simulink model "sistema_nastro_trasportatore"  (R2017a)
settings: Solver=VariableStepAuto  StartTime=0.0  StopTime=10.0  RelTol=1e-3
values from neighbouring files (symbols this model uses):
  A = ro*area    (= 1500)    [params.m]
  B = Ks/A    (= 0.5)    [params.m]
  C = 1    [params.m]
  Km = 1/Y_MAX    (= 0.1)    [params.m]
  r = 0.5    [params.m]
  T = 0.1    [params.m]
  tau = 0.6    [params.m]
libraries: simulink x3
settings Model: Creator=Lucario95  LastModifiedBy=Lucario95

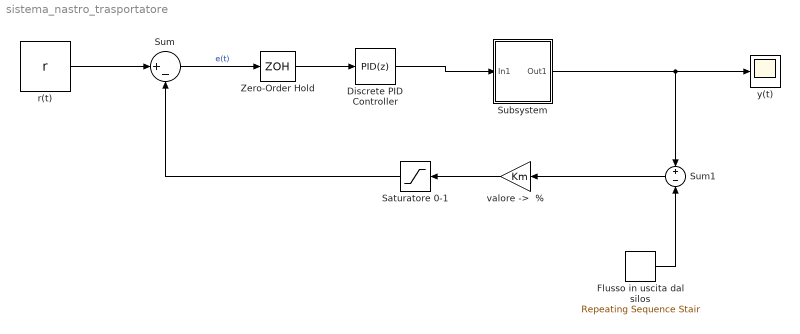
== system sistema_nastro_trasportatore ==
  Discrete PID Controller : simulink/Continuous/PID Controller  Controller=PID  TimeDomain=Discrete-time  SampleTime=-1  IntegratorMethod=Forward Euler  FilterMethod=Forward Euler  Form=Parallel  UseFilter=on  ControllerParametersSource=internal  P=1  I=1  D=0  N=100  InitialConditionSource=internal  InitialConditionForIntegrator=0  InitialConditionForFilter=0  ExternalReset=none  LimitOutput=off  UpperSaturationLimit=inf  LowerSaturationLimit=-inf  LinearizeAsGain=off  AntiWindupMode=none  Kb=1  TrackingMode=off  Kt=1  PParamMin=[]  PParamMax=[]  IParamMin=[]  IParamMax=[]  DParamMin=[]  DParamMax=[]  NParamMin=[]  NParamMax=[]  KbParamMin=[]  KbParamMax=[]  KtParamMin=[]  KtParamMax=[]  POutMin=[]  POutMax=[]  IOutMin=[]  IOutMax=[]  DOutMin=[]  DOutMax=[]  NOutMin=[]  NOutMax=[]  KbOutMin=[]  KbOutMax=[]  KtOutMin=[]  KtOutMax=[]  IntegratorOutMin=[]  IntegratorOutMax=[]  FilterOutMin=[]  FilterOutMax=[]  SumOutMin=[]  SumOutMax=[]  SumI1OutMin=[]  SumI1OutMax=[]  SumI2OutMin=[]  SumI2OutMax=[]  SumI3OutMin=[]  SumI3OutMax=[]  SumDOutMin=[]  SumDOutMax=[]  SaturationOutMin=[]  SaturationOutMax=[]  IntegratorContinuousStateAttributes=''  IntegratorStateMustResolveToSignalObject=off  IntegratorRTWStateStorageClass=Auto  FilterContinuousStateAttributes=''  FilterStateMustResolveToSignalObject=off  FilterRTWStateStorageClass=Auto  DifferentiatorICPrevScaledInput=0  DifferentiatorOutMin=[]  DifferentiatorOutMax=[]  InitialConditionSetting=State (most efficient)
  "Flusso in uscita dal silos " : simulink/Sources/Repeating Sequence Stair  OutValues=[3 1 4 2 1].'  tsamp=T  OutMin=[]  OutMax=[]  OutDataTypeStr=double  OutputDataTypeScalingMode=double  OutDataType=fixdt(0,8)  ConRadixGroup=Best Precision: Vector-wise  OutScaling=2^-12
  "Saturatore 0-1 " : Saturate  UpperLimit=1  LowerLimit=0
  Subsystem : Subsystem
  Sum : Sum  Inputs=|+-
  Sum1 : Sum  Inputs=+-
  Zero-Order Hold : ZeroOrderHold  SampleTime=T
  "r(t) " : Constant  Value=r
  "valore ->  % " : Gain  Gain=Km
  "y(t) " : Scope
  wires:
  "r(t) "/1 -> Sum/1
  Sum/1 -> Zero-Order Hold/1  "e(t)"
  Zero-Order Hold/1 -> Discrete PID Controller/1
  "valore ->  % "/1 -> "Saturatore 0-1 "/1
  "Saturatore 0-1 "/1 -> Sum/2
  Subsystem/1(Out1) -> "y(t) "/1, Sum1/1
  Discrete PID Controller/1 -> Subsystem/1(In1)
  Sum1/1 -> "valore ->  % "/1
  "Flusso in uscita dal silos "/1 -> Sum1/2

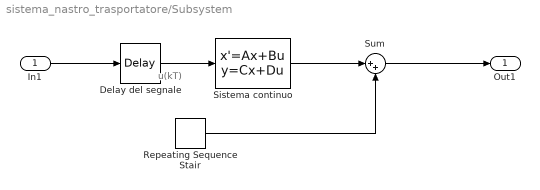
== system sistema_nastro_trasportatore/Subsystem ==
  note: u(kT)
  In1 : Inport
  "Delay del segnale " : TransportDelay  DelayTime=tau
  Repeating Sequence Stair : simulink/Sources/Repeating Sequence Stair  OutValues=[3 1 4 2 1].'  tsamp=T  OutMin=[]  OutMax=[]  OutDataTypeStr=double  OutputDataTypeScalingMode=double  OutDataType=fixdt(0,8)  ConRadixGroup=Best Precision: Vector-wise  OutScaling=2^-12
  "Sistema continuo " : StateSpace  A=A  B=B  C=C  D=0  X0=0
  Sum : Sum  Inputs=|++
  Out1 : Outport
  wires:
  "Delay del segnale "/1 -> "Sistema continuo "/1
  In1/1 -> "Delay del segnale "/1
  Repeating Sequence Stair/1 -> Sum/2
  "Sistema continuo "/1 -> Sum/1
  Sum/1 -> Out1/1
